simulink model "lab2"  (R2015b)
settings: Solver=ode45  StartTime=0.0  StopTime=50  RelTol=1e-3
undefined symbols (not defined in the file or in its folder): serial
libraries: instrumentlib x3
settings Model: Creator=user  LastModifiedBy=ovi
settings DataIOCC: SaveFormat=Array
settings DebuggingCC: UnderspecifiedInitializationDetection=Classic  MergeDetectMultiDrivingBlocksExec=none  SolverPrmCheckMsg=warning  StateNameClashWarn=warning
settings HardwareCC: ProdBitPerPointer=32  ProdLargestAtomicFloat=None  ProdIntDivRoundTo=Undefined  ProdEndianess=Unspecified  ProdWordSize=32  ProdHWDeviceType=32-bit Generic
settings GRTTargetCC: GeneratePreprocessorConditionals=Disable all
settings ConfigComp: CovModelRefEnable=Off

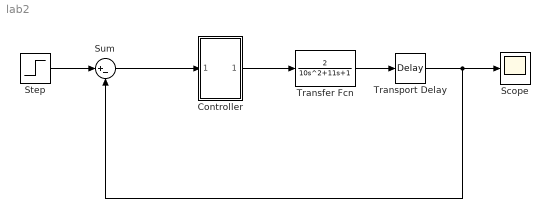
== system lab2 ==
  Controller : Subsystem
  Scope : Scope
  Step : Step  SampleTime=0
  Sum : Sum  Inputs=|+-
  Transfer Fcn : TransferFcn  Numerator=[2]  Denominator=[10 11 1]
  Transport Delay : TransportDelay
  wires:
  Sum/1 -> Controller/1(In1)
  Controller/1(Out1) -> Transfer Fcn/1
  Transport Delay/1 -> Sum/2, Scope/1
  Transfer Fcn/1 -> Transport Delay/1
  Step/1 -> Sum/1

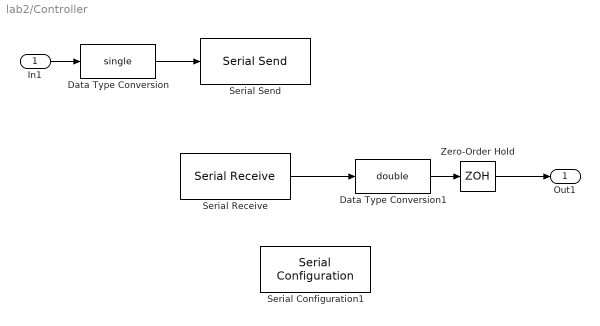
== system lab2/Controller ==
  In1 : Inport
  Data Type Conversion : DataTypeConversion  OutDataTypeStr=single  SampleTime=0.1
  Data Type Conversion1 : DataTypeConversion  OutDataTypeStr=double  SampleTime=0.1
  Serial Configuration1 : instrumentlib/Serial Configuration  Priority=-200000  ComPortMenu=/dev/cu.usbmodem14201  ComPort=/dev/cu.usbmodem14201  ObjConstructor=serial('/dev/cu.usbmodem14201');  BaudRate=9600  DataBits=8  Parity=none  StopBits=1  FlowControl=none  Timeout=10  ByteOrder=LittleEndian
  Serial Receive : instrumentlib/Serial Receive  ComPortMenu=/dev/cu.usbmodem14201  ComPort=/dev/cu.usbmodem14201  ObjConstructor=serial('/dev/cu.usbmodem14201');  Terminator=<none>  DataSize=[1 1]  DataType=uint8  EnableBlockingMode=on  ActionDataUnavailable=Output last received value  CustomValue=0  SampleTime=0.1
  Serial Send : instrumentlib/Serial Send  ComPortMenu=/dev/cu.usbmodem14201  ComPort=/dev/cu.usbmodem14201  ObjConstructor=serial('/dev/cu.usbmodem14201');  Terminator=<none>  EnableBlockingMode=on
  Zero-Order Hold : ZeroOrderHold  SampleTime=0.1
  Out1 : Outport
  wires:
  In1/1 -> Data Type Conversion/1
  Serial Receive/1 -> Data Type Conversion1/1
  Data Type Conversion/1 -> Serial Send/1
  Data Type Conversion1/1 -> Zero-Order Hold/1
  Zero-Order Hold/1 -> Out1/1
